simulink model "playground"  (R2020a)
settings: Solver=VariableStepAuto  StartTime=0  StopTime=30  FixedStep=0.1  MaxStep=0.1  RelTol=1e-3
settings Model: Creator=Peter  LastModifiedBy=Peter

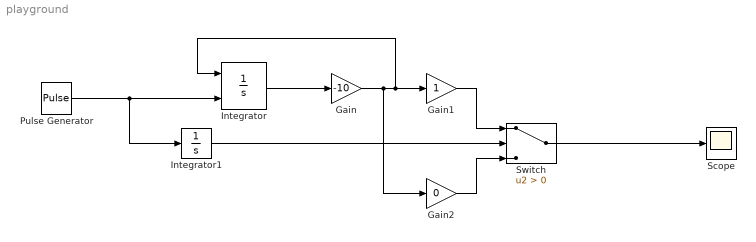
== system playground ==
  Gain : Gain  Gain=-10
  Gain1 : Gain
  Gain2 : Gain  Gain=0
  Integrator : Integrator  ExternalReset=rising  InitialCondition=-1
  Integrator1 : Integrator
  Pulse Generator : DiscretePulseGenerator  PulseType=Time based  Period=5  PulseWidth=50  PhaseDelay=10
  Scope : Scope
  Switch : Switch  Criteria=u2 > Threshold
  wires:
  Integrator/1 -> Gain/1
  Gain/1 -> Gain2/1, Gain1/1, Integrator/1
  Pulse Generator/1 -> Integrator1/1, Integrator/2
  Integrator1/1 -> Switch/2
  Gain1/1 -> Switch/1
  Gain2/1 -> Switch/3
  Switch/1 -> Scope/1
